simulink model "MPC_new"  (R2018b)
settings: Solver=VariableStepAuto  StartTime=0.0  StopTime=Inf  FixedStep=T  RelTol=1e-3
PostLoadFcn:
  | , if any(exist('dsrtsu_mdlpostloadfcn', 'file') ~= 0), dsrtsu_mdlpostloadfcn('Execute', bdroot); end,
values from neighbouring files (symbols this model uses):
  fixed_io_gain = 175    [parameters.m]
  fixed_vclamp_gain = 1000    [parameters.m]
  fixed_vi_gain = 5800    [parameters.m]
  ioa_gain = 1    [parameters.m]
  ioa_offset = -39.5    [parameters.m]
  iob_gain = 1    [parameters.m]
  iob_offset = -39.9    [parameters.m]
  ioc_gain = 1    [parameters.m]
  ioc_offset = -39.34    [parameters.m]
  L = 13.5e-3    (= 0.0135)    [parameters.m]
  R = 10    [parameters.m]
  T = 10*2*2e-6    (= 4e-05)    [parameters.m]
  threshold = 80    [parameters.m]
  vclamp_gain = 1    [parameters.m]
  vclamp_offset = -0.9    [parameters.m]
  via_gain = 1    [parameters.m]
  via_offset = -836.4    [parameters.m]
  vib_gain = 1    [parameters.m]
  vib_offset = -854.9    [parameters.m]
  vic_gain = 1    [parameters.m]
  vic_offset = -852.3    [parameters.m]
undefined symbols (not defined in the file or in its folder): S
libraries: xbsIndex_r4 x416, rti1202lib_adc_class1 x8, rtiproclib x5, simulink x3, rtifpgainterfacelib x1
(part 7 of 7)

== system MPC_new/FPGA_fourstep/FPGA_IO_WRITE_BL9/dig_inout_tp1 ==
  note: The Digital In value is simulated by Threshold voltage detection.
  note: The nominal input range is NOT simulated because
      | the HW does not saturate according to the input range.
  data_in_i : Inport
  enable_i : Inport  Port=2
  data_out_i : Inport  Port=3
  direction_i : Inport  Port=4
  Data Type Conversion : DataTypeConversion
  Data Type Conversion1 : DataTypeConversion
  Disabled Input Value : Constant  Value=0
  Disabled Output Value : Constant  Value=0
  Invert : Constant  Value=inverted_dio
  Invert1 : Constant  Value=inverted_dio
  Inverter : Logic  Operator=NOT  AllPortsSameDT=off  OutDataTypeStr=boolean
  Inverter1 : Logic  AllPortsSameDT=off  OutDataTypeStr=boolean
  Inverter2 : Logic  Operator=NOT  AllPortsSameDT=off  OutDataTypeStr=boolean
  Inverter3 : Logic  AllPortsSameDT=off  OutDataTypeStr=boolean
  Inverter4 : Logic  Operator=NOT  AllPortsSameDT=off  OutDataTypeStr=boolean
  Relational Operator : RelationalOperator  OutDataTypeStr=boolean  RndMeth=Nearest
  Switch{,1..3} (4 alike) : Switch  Threshold=1
  Threshold Voltage : Constant  Value=2
  Voltage : Gain  Gain=voltage  ParamDataTypeStr=float('double')
  data_in_o : Outport
  data_out_o : Outport  Port=2
  wires:
  data_in_i/1 -> Relational Operator/1
  Threshold Voltage/1 -> Relational Operator/2
  Disabled Input Value/1 -> Switch/3
  Switch1/1 -> data_in_o/1
  Invert/1 -> Switch1/2
  Inverter/1 -> Switch1/1
  Relational Operator/1 -> Switch/1
  Switch/1 -> Inverter/1, Switch1/3
  enable_i/1 -> Data Type Conversion/1
  Inverter1/1 -> Switch/2
  direction_i/1 -> Data Type Conversion1/1
  Inverter2/1 -> Inverter1/2
  Disabled Output Value/1 -> Switch2/3
  Inverter3/1 -> Switch2/2
  data_out_i/1 -> Switch2/1
  Invert1/1 -> Switch3/2
  Inverter4/1 -> Switch3/1
  Switch2/1 -> Inverter4/1, Switch3/3
  Switch3/1 -> Voltage/1
  Data Type Conversion/1 -> Inverter1/1, Inverter3/1
  Data Type Conversion1/1 -> Inverter2/1, Inverter3/2
  Voltage/1 -> data_out_o/1

== system MPC_new/FPGA_fourstep/FPGA_XDATA_READ_BL1/phs_read_register ==
  note: Subsystem simulating the communication
      | function specific behaviour. This is how the
      | FPGA framework driver takes effect on the data.
  note: Subsystem simulating the phs bus
      | access via RTLib functions.
  data_i : Inport
  com_fct_model : Subsystem
  phs/rtlib_sim_model : Subsystem
  data_o : Outport
  data_new_o : Outport  Port=2
  wires:
  data_i/1 -> phs/rtlib_sim_model/1(data_i1)
  com_fct_model/1(data_o1) -> data_o/1
  phs/rtlib_sim_model/1(data_o1) -> com_fct_model/1(data_i1)
  com_fct_model/2(data_new_o) -> data_new_o/1

== system MPC_new/FPGA_fourstep/FPGA_XDATA_READ_BL2/phs_read_register ==
  note: Subsystem simulating the communication
      | function specific behaviour. This is how the
      | FPGA framework driver takes effect on the data.
  note: Subsystem simulating the phs bus
      | access via RTLib functions.
  data_i : Inport
  com_fct_model : Subsystem
  phs/rtlib_sim_model : Subsystem
  data_o : Outport
  data_new_o : Outport  Port=2
  wires:
  data_i/1 -> phs/rtlib_sim_model/1(data_i1)
  com_fct_model/1(data_o1) -> data_o/1
  phs/rtlib_sim_model/1(data_o1) -> com_fct_model/1(data_i1)
  com_fct_model/2(data_new_o) -> data_new_o/1

== system MPC_new/FPGA_fourstep/FPGA_XDATA_READ_BL3/phs_read_register ==
  note: Subsystem simulating the communication
      | function specific behaviour. This is how the
      | FPGA framework driver takes effect on the data.
  note: Subsystem simulating the phs bus
      | access via RTLib functions.
  data_i : Inport
  com_fct_model : Subsystem
  phs/rtlib_sim_model : Subsystem
  data_o : Outport
  data_new_o : Outport  Port=2
  wires:
  data_i/1 -> phs/rtlib_sim_model/1(data_i1)
  com_fct_model/1(data_o1) -> data_o/1
  phs/rtlib_sim_model/1(data_o1) -> com_fct_model/1(data_i1)
  com_fct_model/2(data_new_o) -> data_new_o/1

== system MPC_new/RTI Data/RTI Data Store/RTI Data Store ==
  RTI Data Store : Subsystem  mask(RTI_DATA_STORE){}
      mask help:
      | RTI Data Store Block. This block is used by RTI to store internal model dependent data. Deleting this block will result in data loss.
      |
      | NEVER DELETE, COPY, OR MODIFY THIS BLOCK!
      mask Help:
      | RTI Data Store Block. This block is used by RTI to store internal model dependent data. Deleting this block will result in data loss.
      | 
      | NEVER DELETE, COPY, OR MODIFY THIS BLOCK!
      mask Display: text(0.5, 0.5, ' ', 'HorizontalAlignment', 'center');

== system MPC_new/FPGA_fourstep/FPGA_INT_BL1/phs_interrupt/com_fct_model ==
  data_i1 : Inport
  data_o1 : Outport
  wires:
  data_i1/1 -> data_o1/1

== system MPC_new/FPGA_fourstep/FPGA_INT_BL1/phs_interrupt/phs//rtlib_sim_model ==
  note: - Detect the interrupt (rising edge).
      | - Generate function call.
  data_i1 : Inport
  Triggered Subsystem : Subsystem  TreatAsAtomicUnit=on
  data_o1 : Outport
  wires:
  data_i1/1 -> Triggered Subsystem/Trigger
  Triggered Subsystem/1(Out1) -> data_o1/1

== system MPC_new/FPGA_fourstep/FPGA_XDATA_READ_BL1/phs_read_register/com_fct_model ==
  note: - Register data is presented to the FPGA application without data adaptions.
      |
      | - Register group accesses are implicitly simulated by simulink: all FPGA
      | communication function interface blocks are simulated within one task
      | with a unique sample time --> in- and ouputs are sampled simultaneously
      | and therefore data consistency is guaranteed.
  data_i1 : Inport
  Data_New_Calc : Subsystem
  Zero-Order Hold : ZeroOrderHold  SampleTime=fpga_sample_time
  data_o1 : Outport
  data_new_o : Outport  Port=2
  wires:
  data_i1/1 -> Data_New_Calc/1(In1), Zero-Order Hold/1
  Data_New_Calc/1(Out1) -> data_new_o/1
  Zero-Order Hold/1 -> data_o1/1

== system MPC_new/FPGA_fourstep/FPGA_XDATA_READ_BL1/phs_read_register/phs//rtlib_sim_model ==
  note: - The double to fixed-point conversion done by the XSG gateway behaves differently
      | than the conversion done by the RTLib C-code. Therefore the C-Code behaviour
      | is simulated via an s-function using the RTLib conversion technique including scaling and saturation.
  data_i1 : Inport
  S-Function : S-Function  FunctionName=DS1302_read_register  Parameters=mode;binaryPoint  SFunctionDeploymentMode=off  EnableBusSupport=off
  Zero-Order Hold : ZeroOrderHold  SampleTime=proc_sample_time
  data_o1 : Outport
  wires:
  data_i1/1 -> Zero-Order Hold/1
  S-Function/1 -> data_o1/1
  Zero-Order Hold/1 -> S-Function/1

== system MPC_new/FPGA_fourstep/FPGA_XDATA_READ_BL2/phs_read_register/com_fct_model ==
  note: - Register data is presented to the FPGA application without data adaptions.
      |
      | - Register group accesses are implicitly simulated by simulink: all FPGA
      | communication function interface blocks are simulated within one task
      | with a unique sample time --> in- and ouputs are sampled simultaneously
      | and therefore data consistency is guaranteed.
  data_i1 : Inport
  Data_New_Calc : Subsystem
  Zero-Order Hold : ZeroOrderHold  SampleTime=fpga_sample_time
  data_o1 : Outport
  data_new_o : Outport  Port=2
  wires:
  data_i1/1 -> Data_New_Calc/1(In1), Zero-Order Hold/1
  Data_New_Calc/1(Out1) -> data_new_o/1
  Zero-Order Hold/1 -> data_o1/1

== system MPC_new/FPGA_fourstep/FPGA_XDATA_READ_BL2/phs_read_register/phs//rtlib_sim_model ==
  note: - The double to fixed-point conversion done by the XSG gateway behaves differently
      | than the conversion done by the RTLib C-code. Therefore the C-Code behaviour
      | is simulated via an s-function using the RTLib conversion technique including scaling and saturation.
  data_i1 : Inport
  S-Function : S-Function  FunctionName=DS1302_read_register  Parameters=mode;binaryPoint  SFunctionDeploymentMode=off  EnableBusSupport=off
  Zero-Order Hold : ZeroOrderHold  SampleTime=proc_sample_time
  data_o1 : Outport
  wires:
  data_i1/1 -> Zero-Order Hold/1
  S-Function/1 -> data_o1/1
  Zero-Order Hold/1 -> S-Function/1

== system MPC_new/FPGA_fourstep/FPGA_XDATA_READ_BL3/phs_read_register/com_fct_model ==
  note: - Register data is presented to the FPGA application without data adaptions.
      |
      | - Register group accesses are implicitly simulated by simulink: all FPGA
      | communication function interface blocks are simulated within one task
      | with a unique sample time --> in- and ouputs are sampled simultaneously
      | and therefore data consistency is guaranteed.
  data_i1 : Inport
  Data_New_Calc : Subsystem
  Zero-Order Hold : ZeroOrderHold  SampleTime=fpga_sample_time
  data_o1 : Outport
  data_new_o : Outport  Port=2
  wires:
  data_i1/1 -> Data_New_Calc/1(In1), Zero-Order Hold/1
  Data_New_Calc/1(Out1) -> data_new_o/1
  Zero-Order Hold/1 -> data_o1/1

== system MPC_new/FPGA_fourstep/FPGA_XDATA_READ_BL3/phs_read_register/phs//rtlib_sim_model ==
  note: - The double to fixed-point conversion done by the XSG gateway behaves differently
      | than the conversion done by the RTLib C-code. Therefore the C-Code behaviour
      | is simulated via an s-function using the RTLib conversion technique including scaling and saturation.
  data_i1 : Inport
  S-Function : S-Function  FunctionName=DS1302_read_register  Parameters=mode;binaryPoint  SFunctionDeploymentMode=off  EnableBusSupport=off
  Zero-Order Hold : ZeroOrderHold  SampleTime=proc_sample_time
  data_o1 : Outport
  wires:
  data_i1/1 -> Zero-Order Hold/1
  S-Function/1 -> data_o1/1
  Zero-Order Hold/1 -> S-Function/1

== system MPC_new/RTI Data/RTI Data Store/RTI Data Store/RTI Data Store ==
  RTI Data Store : Subsystem  mask(RTI_DATA_STORE){}
      mask help:
      | RTI Data Store Block. This block is used by RTI to store internal model dependent data. Deleting this block will result in data loss.
      |
      | NEVER DELETE, COPY, OR MODIFY THIS BLOCK!
      mask Help:
      | RTI Data Store Block. This block is used by RTI to store internal model dependent data. Deleting this block will result in data loss.
      | 
      | NEVER DELETE, COPY, OR MODIFY THIS BLOCK!
      mask Display: text(0.5, 0.5, ' ', 'HorizontalAlignment', 'center');

== system MPC_new/FPGA_fourstep/FPGA_INT_BL1/phs_interrupt/phs//rtlib_sim_model/Triggered Subsystem ==
  Trigger : TriggerPort  VariantControl=(inherit)
  Function-Call Generator : simulink/Ports & Subsystems/Function-Call Generator  sample_time=-1  numberOfIterations=1
  Out1 : Outport
  wires:
  Function-Call Generator/1 -> Out1/1

== system MPC_new/FPGA_fourstep/FPGA_XDATA_READ_BL1/phs_read_register/com_fct_model/Data_New_Calc ==
  note: The new data flag is presented whenever the input data port is sampled.
      | The flag is set to 1 for one FPGA simulation step and reset to 0 for the
      | remaining FPGA simulation steps contained within one processor simulation step.
  In1 : Inport
  Add : Sum
  Constant : Constant  Value=fpga_sample_time  SampleTime=fpga_sample_time
  Constant1 : Constant  Value=0
  Divide : Product  Inputs=*/
  Divide1 : Product  Inputs=*/
  Math Function : Math  Operator=mod  SaturateOnIntegerOverflow=on
  Relational Operator : RelationalOperator  Operator===  OutDataTypeStr=boolean  RndMeth=Nearest
  Unit Delay1 : UnitDelay  InitialCondition=-1  SampleTime=-1
  Weighted Sample Time1 : SampleTimeMath  TsampMathOp=Ts Only
  Out1 : Outport
  wires:
  Divide/1 -> Math Function/2
  Constant1/1 -> Relational Operator/2
  Add/1 -> Math Function/1, Unit Delay1/1
  Unit Delay1/1 -> Add/2
  Divide1/1 -> Add/1
  In1/1 -> Weighted Sample Time1/1
  Relational Operator/1 -> Out1/1
  Math Function/1 -> Relational Operator/1
  Weighted Sample Time1/1 -> Divide/1
  Constant/1 -> Divide/2, Divide1/1, Divide1/2

== system MPC_new/FPGA_fourstep/FPGA_XDATA_READ_BL2/phs_read_register/com_fct_model/Data_New_Calc ==
  note: The new data flag is presented whenever the input data port is sampled.
      | The flag is set to 1 for one FPGA simulation step and reset to 0 for the
      | remaining FPGA simulation steps contained within one processor simulation step.
  In1 : Inport
  Add : Sum
  Constant : Constant  Value=fpga_sample_time  SampleTime=fpga_sample_time
  Constant1 : Constant  Value=0
  Divide : Product  Inputs=*/
  Divide1 : Product  Inputs=*/
  Math Function : Math  Operator=mod  SaturateOnIntegerOverflow=on
  Relational Operator : RelationalOperator  Operator===  OutDataTypeStr=boolean  RndMeth=Nearest
  Unit Delay1 : UnitDelay  InitialCondition=-1  SampleTime=-1
  Weighted Sample Time1 : SampleTimeMath  TsampMathOp=Ts Only
  Out1 : Outport
  wires:
  Divide/1 -> Math Function/2
  Constant1/1 -> Relational Operator/2
  Add/1 -> Math Function/1, Unit Delay1/1
  Unit Delay1/1 -> Add/2
  Divide1/1 -> Add/1
  In1/1 -> Weighted Sample Time1/1
  Relational Operator/1 -> Out1/1
  Math Function/1 -> Relational Operator/1
  Weighted Sample Time1/1 -> Divide/1
  Constant/1 -> Divide/2, Divide1/1, Divide1/2

== system MPC_new/FPGA_fourstep/FPGA_XDATA_READ_BL3/phs_read_register/com_fct_model/Data_New_Calc ==
  note: The new data flag is presented whenever the input data port is sampled.
      | The flag is set to 1 for one FPGA simulation step and reset to 0 for the
      | remaining FPGA simulation steps contained within one processor simulation step.
  In1 : Inport
  Add : Sum
  Constant : Constant  Value=fpga_sample_time  SampleTime=fpga_sample_time
  Constant1 : Constant  Value=0
  Divide : Product  Inputs=*/
  Divide1 : Product  Inputs=*/
  Math Function : Math  Operator=mod  SaturateOnIntegerOverflow=on
  Relational Operator : RelationalOperator  Operator===  OutDataTypeStr=boolean  RndMeth=Nearest
  Unit Delay1 : UnitDelay  InitialCondition=-1  SampleTime=-1
  Weighted Sample Time1 : SampleTimeMath  TsampMathOp=Ts Only
  Out1 : Outport
  wires:
  Divide/1 -> Math Function/2
  Constant1/1 -> Relational Operator/2
  Add/1 -> Math Function/1, Unit Delay1/1
  Unit Delay1/1 -> Add/2
  Divide1/1 -> Add/1
  In1/1 -> Weighted Sample Time1/1
  Relational Operator/1 -> Out1/1
  Math Function/1 -> Relational Operator/1
  Weighted Sample Time1/1 -> Divide/1
  Constant/1 -> Divide/2, Divide1/1, Divide1/2

== system MPC_new/RTI Data/RTI Data Store/RTI Data Store/RTI Data Store/RTI Data Store ==

== matlab function MPC_new/datatype_conversion ==
  data: u input; y output
function y = v2dec(u)

y = u(1)+2*u(2)+4*u(3);

== matlab function MPC_new/control/MATLAB Function ==
  data: io input; out output; iref input; vi input; S input; R input; L input; T input
function out  = MPC_func(io, iref, vi, S, R, L, T)
kopt = 19;
mincost = 100000000;
i_med = io;
v_med = vi;
ir = iref;

for k = 1:27
    v = S(:,:,k)*v_med;
    i = (1 - R*T/L)*i_med + (T/L)*v;
    e = ir - i;
    cost = e'*e;
    if cost <= mincost
        kopt = k;
        mincost = cost;
    end
end
out = kopt;
end
